simulink model "NEW_NL0_NEW1"  (R2024a)
settings: Solver=VariableStepAuto  StartTime=0.0  StopTime=100  FixedStep=0.0001  MaxStep=1e-2  MinStep=1e-12  RelTol=1e-6  AbsTol=1e-6
libraries: fl_lib x15, nesl_utility x6, simulink x1, sdl_lib x1
settings Model: Creator=yl14470  LastModifiedBy=sa21280
settings RTWCC: GPUComputeCapability=3.5

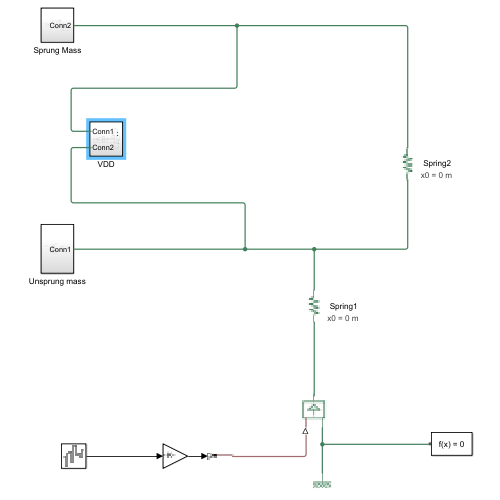
[thumbnail: Simulink's stored preview of the top-level diagram]
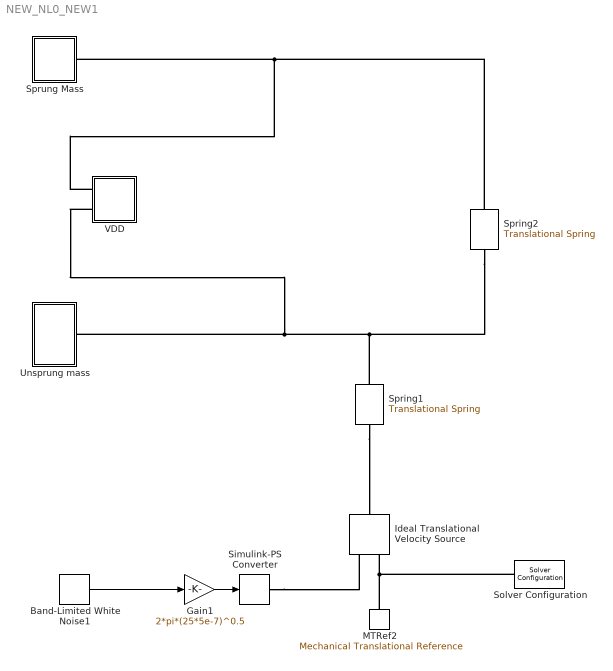
== system NEW_NL0_NEW1 ==
  Band-Limited White Noise1 : simulink/Sources/Band-Limited White Noise  Cov=1  Ts=0.0001  seed=[23341]
  Gain1 : Gain  Gain=2*pi*(25*5e-7)^0.5
  Ideal Translational Velocity Source : fl_lib/Mechanical/Mechanical Sources/Ideal Translational Velocity Source
  MTRef2 : fl_lib/Mechanical/Translational Elements/Mechanical Translational Reference
  Simulink-PS Converter : nesl_utility/Simulink-PS Converter  PhysicalDomain=network_engine_domain  SubClassName=ps_input  LeftPortType=input  RightPortType=output  PseudoPeriodic=off  Frequencies=[]  NoiseDistribution=none  NoiseParameters=[]  Unit=m/s  AffineConversion=off  FilteringAndDerivatives=filter  SimscapeFilterOrder=1  InputFilterTimeConstant=0.001  UdotUserProvided=0
  Solver Configuration : nesl_utility/Solver Configuration  PhysicalDomain=network_engine_domain  SubClassName=solver  LeftPortType=input  RightPortType=generic  Tones=[]  Harmonics=[]  SimulateNoise=off  Profile=off  UseLocalSampling=off  EnableSwitchedLinearOptims=on  FrequencyDomain=off  UseCCode=off  RelTol=0.001  AbsTol=1e-06  MinStep=1e-09  ToWorkspace=off  RevertToSquareIcSolve=off  NumHomotopyIterations=100  PhasorMode=off  PhasorModeNumHarmonics=1  ConsistencySolver=NEWTON_FTOL  IndexReductionMethod=DerivativeReplacement  DoDC=off  ResidualTolerance=1e-9  ConsistencyTolSource=GLOBAL  ConsistencyAbsTol=0.001  ConsistencyRelTol=0.001  ConsistencyTolFactor=0.001  UseLocalSolver=off  LocalSolverChoice=NE_BACKWARD_EULER_ADVANCER  ResolveIndetEquations=on  FunctionEvalNumThread=1  LocalSolverSampleTime=.001  DoFixedCost=off  MaxNonlinIter=12  MaxModeIter=2  ComputeImpulses=off  ImpulseIterations=2  LinearAlgebra=Sparse  LinearAlgebraNumThread=0  EquationFormulation=NE_TIME_EF  DelaysMemoryBudget=1024  AutomaticFiltering=on  FilteringTimeConstant=0.001  PartitionStorageMethod=AS_NEEDED  PartitionMemoryBudget=1024  PartitionMethod=FAST  MultibodyUseLocalSolver=off  MultibodyLocalSolverChoice=ODE1  MultibodyLocalSolverSampleTime=0.001
  Spring1 : fl_lib/Mechanical/Translational Elements/Translational Spring  spr_rate=160000 N/m  v_specify=off  v_priority=High  v=0 m/s  v_nominal_specify=off  v_nominal_value=1  v_nominal_unit=m/s  f_specify=off  f_priority=High  f=0 N  f_nominal_specify=off  f_nominal_value=1  f_nominal_unit=N  x_specify=on  x_priority=High  x=0 m  x_nominal_specify=off  x_nominal_value=1  x_nominal_unit=m
      settings: AttributesFormatString=x0 = %<x> %<x_unit>
  Spring2 : fl_lib/Mechanical/Translational Elements/Translational Spring  spr_rate=16998.2107 N/m  v_specify=off  v_priority=High  v=0 m/s  v_nominal_specify=off  v_nominal_value=1  v_nominal_unit=m/s  f_specify=off  f_priority=High  f=0 N  f_nominal_specify=off  f_nominal_value=1  f_nominal_unit=N  x_specify=on  x_priority=High  x=0 m  x_nominal_specify=off  x_nominal_value=1  x_nominal_unit=m
      settings: AttributesFormatString=x0 = %<x> %<x_unit>
  Sprung Mass : Subsystem
  Unsprung mass : Subsystem
  VDD : Subsystem
  wires:
  Gain1/1 -> Simulink-PS Converter/1
  Band-Limited White Noise1/1 -> Gain1/1
  connections:
  Spring1/RConn1 -- Ideal Translational Velocity Source/LConn1
  MTRef2/LConn1 -- Ideal Translational Velocity Source/RConn2 -- Solver Configuration/RConn1
  Simulink-PS Converter/RConn1 -- Ideal Translational Velocity Source/RConn1
  Spring1/LConn1 -- VDD/LConn2 -- Unsprung mass/RConn1 -- Spring2/RConn1
  Spring2/LConn1 -- VDD/LConn1 -- Sprung Mass/RConn1

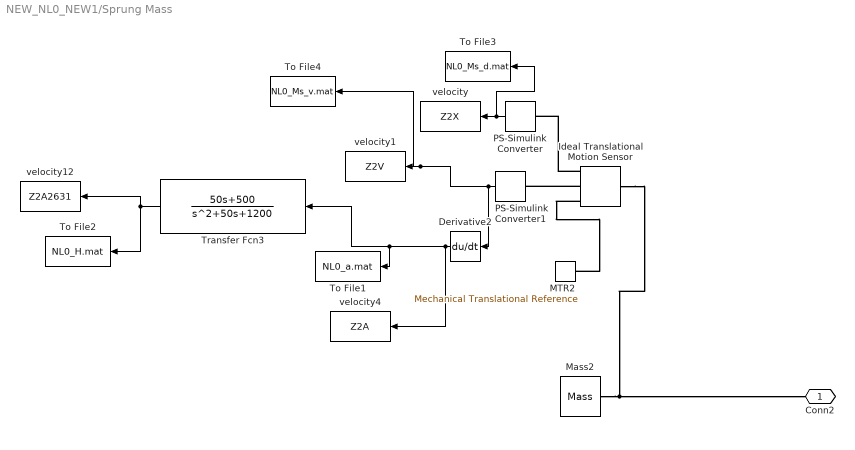
== system NEW_NL0_NEW1/Sprung Mass ==
  Derivative2 : Derivative
  Ideal Translational Motion Sensor : fl_lib/Mechanical/Mechanical Sensors/Ideal Translational Motion Sensor  reference=foundation.enum.MeasurementReference.difference  acceleration_port=false  velocity_port=true  position_port=true  offset=0 m
  MTR2 : fl_lib/Mechanical/Translational Elements/Mechanical Translational Reference
  Mass2 : fl_lib/Mechanical/Translational Elements/Mass  mass=240 kg  num_ports=foundation.enum.numPorts2.one  v_specify=off  v_priority=High  v=0 m/s  v_nominal_specify=off  v_nominal_value=1  v_nominal_unit=m/s  f_specify=off  f_priority=High  f=0 N  f_nominal_specify=off  f_nominal_value=1  f_nominal_unit=N
  PS-Simulink Converter : nesl_utility/PS-Simulink Converter  PhysicalDomain=network_engine_domain  SubClassName=ps_output  LeftPortType=input  RightPortType=output  PseudoPeriodic=off  Frequencies=[]  VectorFormat=1-D array  Unit=1  AffineConversion=off
  PS-Simulink Converter1 : nesl_utility/PS-Simulink Converter  PhysicalDomain=network_engine_domain  SubClassName=ps_output  LeftPortType=input  RightPortType=output  PseudoPeriodic=off  Frequencies=[]  VectorFormat=1-D array  Unit=1  AffineConversion=off
  To File1 : ToFile  Filename=NL0_a.mat  MatrixName=force  SaveFormat=Timeseries
  To File2 : ToFile  Filename=NL0_H.mat  MatrixName=force  SaveFormat=Timeseries
  To File3 : ToFile  Filename=NL0_Ms_d.mat  MatrixName=Ms_d  SaveFormat=Timeseries
  To File4 : ToFile  Filename=NL0_Ms_v.mat  MatrixName=Ms_v  SaveFormat=Timeseries
  Transfer Fcn3 : TransferFcn  Numerator=[0 50 500]  Denominator=[1 50 1200]
  velocity : ToWorkspace  VariableName=Z2X  SampleTime=-1
  velocity1 : ToWorkspace  VariableName=Z2V  SampleTime=-1
  velocity12 : ToWorkspace  VariableName=Z2A2631  SampleTime=-1
  velocity4 : ToWorkspace  VariableName=Z2A  SampleTime=-1
  Conn2 : PMIOPort  Side=Right
  wires:
  Transfer Fcn3/1 -> To File2/1, velocity12/1
  PS-Simulink Converter/1 -> To File3/1, velocity/1
  PS-Simulink Converter1/1 -> Derivative2/1, To File4/1, velocity1/1
  Derivative2/1 -> To File1/1, Transfer Fcn3/1, velocity4/1
  connections:
  Ideal Translational Motion Sensor/RConn1 -- MTR2/LConn1
  Mass2/LConn1 -- Conn2/RConn1 -- Ideal Translational Motion Sensor/LConn1
  Ideal Translational Motion Sensor/RConn2 -- PS-Simulink Converter1/LConn1
  Ideal Translational Motion Sensor/RConn3 -- PS-Simulink Converter/LConn1

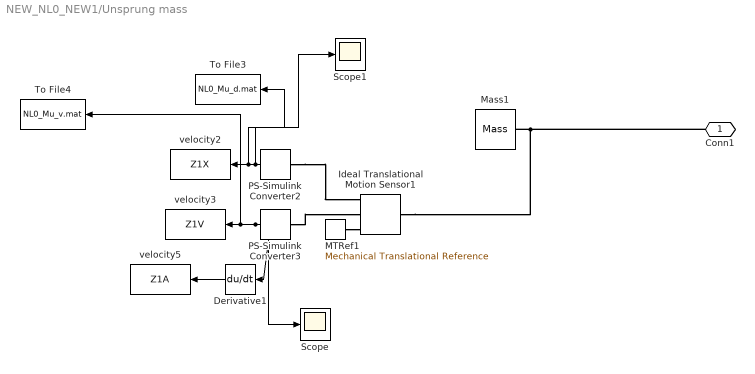
== system NEW_NL0_NEW1/Unsprung mass ==
  Derivative1 : Derivative
  Ideal Translational Motion Sensor1 : fl_lib/Mechanical/Mechanical Sensors/Ideal Translational Motion Sensor  reference=foundation.enum.MeasurementReference.difference  acceleration_port=false  velocity_port=true  position_port=true  offset=0 m
  MTRef1 : fl_lib/Mechanical/Translational Elements/Mechanical Translational Reference
  Mass1 : fl_lib/Mechanical/Translational Elements/Mass  mass=36 kg  num_ports=foundation.enum.numPorts2.one  v_specify=off  v_priority=High  v=0 m/s  v_nominal_specify=off  v_nominal_value=1  v_nominal_unit=m/s  f_specify=off  f_priority=High  f=0 N  f_nominal_specify=off  f_nominal_value=1  f_nominal_unit=N
  PS-Simulink Converter2 : nesl_utility/PS-Simulink Converter  PhysicalDomain=network_engine_domain  SubClassName=ps_output  LeftPortType=input  RightPortType=output  PseudoPeriodic=off  Frequencies=[]  VectorFormat=1-D array  Unit=1  AffineConversion=off
  PS-Simulink Converter3 : nesl_utility/PS-Simulink Converter  PhysicalDomain=network_engine_domain  SubClassName=ps_output  LeftPortType=input  RightPortType=output  PseudoPeriodic=off  Frequencies=[]  VectorFormat=1-D array  Unit=1  AffineConversion=off
  Scope : Scope
  Scope1 : Scope
  To File3 : ToFile  Filename=NL0_Mu_d.mat  MatrixName=Mu_d  SaveFormat=Timeseries
  To File4 : ToFile  Filename=NL0_Mu_v.mat  MatrixName=Mu_v  SaveFormat=Timeseries
  velocity2 : ToWorkspace  VariableName=Z1X  SampleTime=-1
  velocity3 : ToWorkspace  VariableName=Z1V  SampleTime=-1
  velocity5 : ToWorkspace  VariableName=Z1A  SampleTime=-1
  Conn1 : PMIOPort  Side=Right
  wires:
  PS-Simulink Converter3/1 -> To File4/1, velocity3/1, Scope/1, Derivative1/1
  Derivative1/1 -> velocity5/1
  PS-Simulink Converter2/1 -> Scope1/1, To File3/1, velocity2/1
  connections:
  Mass1/LConn1 -- Conn1/RConn1 -- Ideal Translational Motion Sensor1/LConn1
  MTRef1/LConn1 -- Ideal Translational Motion Sensor1/RConn1
  PS-Simulink Converter3/LConn1 -- Ideal Translational Motion Sensor1/RConn2
  PS-Simulink Converter2/LConn1 -- Ideal Translational Motion Sensor1/RConn3

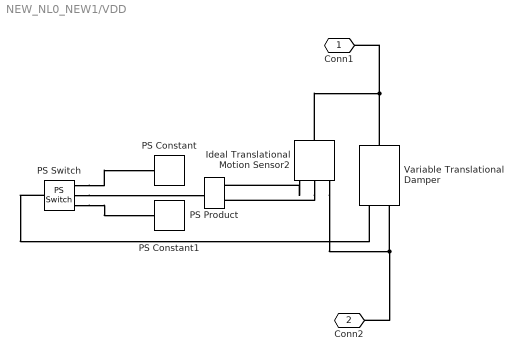
== system NEW_NL0_NEW1/VDD ==
  Ideal Translational Motion Sensor2 : fl_lib/Mechanical/Mechanical Sensors/Ideal Translational Motion Sensor  reference=foundation.enum.MeasurementReference.difference  acceleration_port=false  velocity_port=true  position_port=true  offset=0 m
  PS Constant : fl_lib/Physical Signals/Sources/PS Constant  constant=772 N/(m/s)
  PS Constant1 : fl_lib/Physical Signals/Sources/PS Constant  constant=25.88 N/(m/s)
  PS Product : fl_lib/Physical Signals/Functions/PS Product
  PS Switch : fl_lib/Physical Signals/Nonlinear Operators/PS Switch  Threshold=0 m^2/s
      settings: InternalSimscapePortConfiguration="{\"Bottom\":[],\"Left\":[{\"id\":\"I1\",\"label\":\"\",\"type\":\"input\"},{\"id\":\"I2\",\"label\":\"\",\"type\":\"input\"},{\"id\":\"I3\",\"label\":\"\",\"type\":\"input\"}],\"Right\":[{\"id\":\"O\",\"label\":\"\",\"type\":\"output\"}],\"Top\":[]}"
  Variable Translational Damper : sdl_lib/Couplings & Drives/Springs & Dampers/Variable Translational Damper  Bmin=0 N*s/m
      settings: InternalSimscapePortConfiguration="{\"Bottom\":[],\"Left\":[{\"id\":\"B\",\"label\":\"B\",\"type\":\"input\"},{\"id\":\"R\",\"label\":\"R\",\"type\":\"foundation.mechanical.translational.translational\"}],\"Right\":[{\"id\":\"C\",\"label\":\"C\",\"type\":\"foundation.mechanical.translational.translational\"}],\"Top\":[]}"
  Conn1 : PMIOPort  Side=Left
  Conn2 : PMIOPort  Port=2  Side=Left
  connections:
  PS Switch/LConn2 -- PS Product/RConn1
  Ideal Translational Motion Sensor2/RConn1 -- Conn2/RConn1 -- Variable Translational Damper/LConn2
  Ideal Translational Motion Sensor2/RConn3 -- PS Product/LConn2
  PS Switch/RConn1 -- Variable Translational Damper/LConn1
  Ideal Translational Motion Sensor2/RConn2 -- PS Product/LConn1
  PS Switch/LConn3 -- PS Constant/RConn1
  PS Switch/LConn1 -- PS Constant1/RConn1
  Ideal Translational Motion Sensor2/LConn1 -- Conn1/RConn1 -- Variable Translational Damper/RConn1
